simulink model "fm_rx_model"  (R2021a)
settings: Solver=FixedStepDiscrete  StartTime=0.0  StopTime=2000  FixedStep=1  RelTol=1e-3  EnableMultiTasking=on
settings Model: Creator=user  LastModifiedBy=user
settings DebuggingCC: SingleTaskRateTransMsg=error

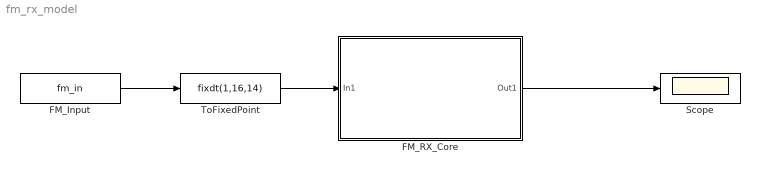
== system fm_rx_model ==
  FM_Input : FromWorkspace  VariableName=fm_in
  FM_RX_Core : Subsystem
  Scope : Scope
  ToFixedPoint : DataTypeConversion  OutDataTypeStr=fixdt(1,16,14)
  wires:
  FM_Input/1 -> ToFixedPoint/1
  ToFixedPoint/1 -> FM_RX_Core/1(In1)
  FM_RX_Core/1(Out1) -> Scope/1

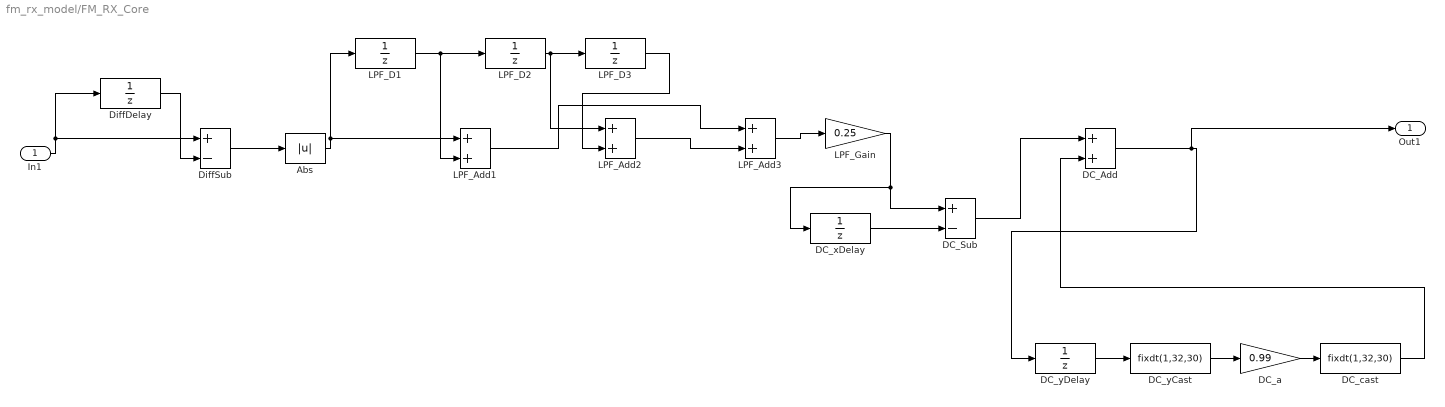
== system fm_rx_model/FM_RX_Core ==
  In1 : Inport
  Abs : Abs
  DC_Add : Sum
  DC_Sub : Sum  Inputs=+-
  DC_a : Gain  Gain=0.99
  DC_cast : DataTypeConversion  OutDataTypeStr=fixdt(1,32,30)
  DC_xDelay : UnitDelay  HasFrameUpgradeWarning=on
  DC_yCast : DataTypeConversion  OutDataTypeStr=fixdt(1,32,30)
  DC_yDelay : UnitDelay  HasFrameUpgradeWarning=on
  DiffDelay : UnitDelay  HasFrameUpgradeWarning=on
  DiffSub : Sum  Inputs=+-
  LPF_Add1 : Sum
  LPF_Add2 : Sum
  LPF_Add3 : Sum
  LPF_D1 : UnitDelay  HasFrameUpgradeWarning=on
  LPF_D2 : UnitDelay  HasFrameUpgradeWarning=on
  LPF_D3 : UnitDelay  HasFrameUpgradeWarning=on
  LPF_Gain : Gain  Gain=0.25
  Out1 : Outport
  wires:
  In1/1 -> DiffDelay/1, DiffSub/1
  DiffDelay/1 -> DiffSub/2
  DiffSub/1 -> Abs/1
  Abs/1 -> LPF_D1/1, LPF_Add1/1
  LPF_D1/1 -> LPF_D2/1, LPF_Add1/2
  LPF_D2/1 -> LPF_D3/1, LPF_Add2/1
  LPF_D3/1 -> LPF_Add2/2
  LPF_Add1/1 -> LPF_Add3/1
  LPF_Add2/1 -> LPF_Add3/2
  LPF_Add3/1 -> LPF_Gain/1
  LPF_Gain/1 -> DC_xDelay/1, DC_Sub/1
  DC_xDelay/1 -> DC_Sub/2
  DC_Sub/1 -> DC_Add/1
  DC_yDelay/1 -> DC_yCast/1
  DC_yCast/1 -> DC_a/1
  DC_a/1 -> DC_cast/1
  DC_cast/1 -> DC_Add/2
  DC_Add/1 -> DC_yDelay/1, Out1/1
